simulink model "p3_1"  (R2018a)
settings: Solver=VariableStepAuto  StartTime=0.0  StopTime=10.0  RelTol=1e-3
settings Model: Creator=ASUS  LastModifiedBy=ASUS

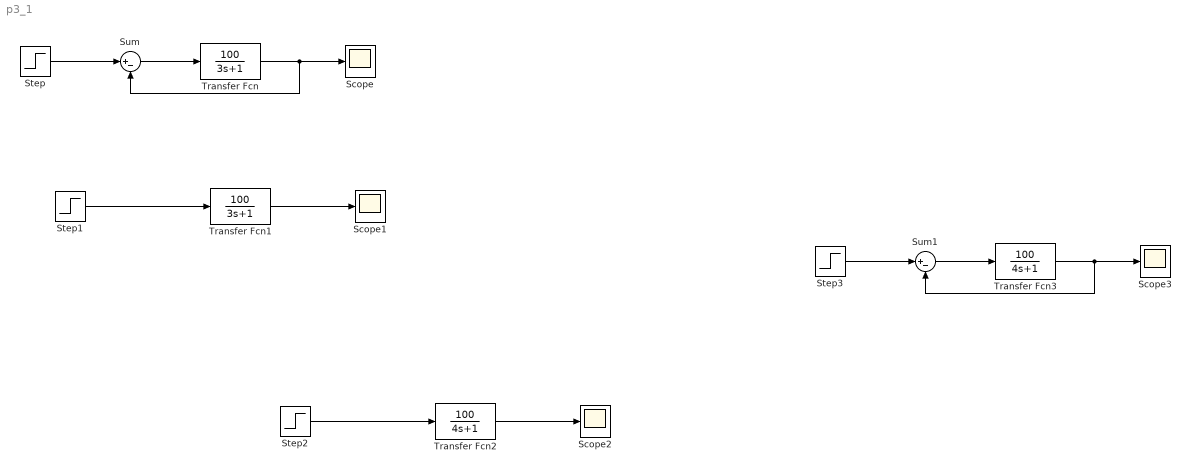
== system p3_1 ==
  Scope{,1..3} (4 alike) : Scope
  Step{,1..3} (4 alike) : Step  Time=0  SampleTime=0
  Sum : Sum  Inputs=|+-
  Sum1 : Sum  Inputs=|+-
  Transfer Fcn : TransferFcn  Numerator=[100]  Denominator=[3 1]
  Transfer Fcn1 : TransferFcn  Numerator=[100]  Denominator=[3 1]
  Transfer Fcn2 : TransferFcn  Numerator=[100]  Denominator=[4 1]
  Transfer Fcn3 : TransferFcn  Numerator=[100]  Denominator=[4 1]
  wires:
  Step/1 -> Sum/1
  Sum/1 -> Transfer Fcn/1
  Transfer Fcn/1 -> Sum/2, Scope/1
  Step1/1 -> Transfer Fcn1/1
  Transfer Fcn1/1 -> Scope1/1
  Step2/1 -> Transfer Fcn2/1
  Transfer Fcn2/1 -> Scope2/1
  Sum1/1 -> Transfer Fcn3/1
  Transfer Fcn3/1 -> Sum1/2, Scope3/1
  Step3/1 -> Sum1/1
